simulink model "fuzzy_system"  (R2017a)
settings: Solver=VariableStepAuto  StartTime=0.0  StopTime=10  RelTol=1e-3
undefined symbols (not defined in the file or in its folder): tanks_level_system
libraries: simulink x1
settings Model: Creator=fredericovaz  LastModifiedBy=fredericovaz
settings SFSimCC: SimUseLocalCustomCode=on
settings RTWCC: RTWUseLocalCustomCode=on

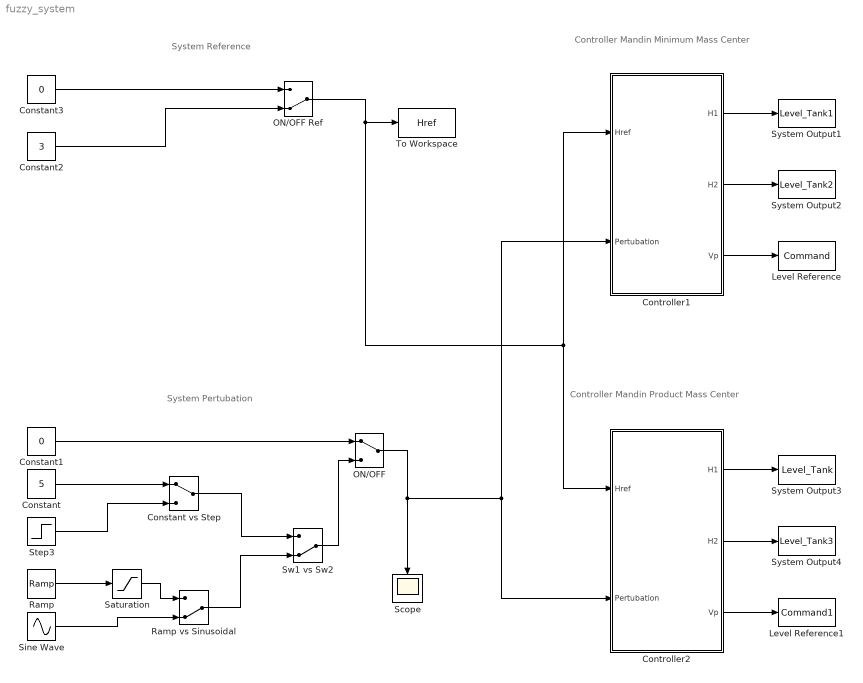
== system fuzzy_system ==
  note: Controller Mandin Minimum Mass Center
  note: Controller Mandin Product Mass Center
  note: System Pertubation
  note: System Reference
  Constant : Constant  Value=5
  Constant vs Step : ManualSwitch
  Constant1 : Constant  Value=0
  Constant2 : Constant  Value=3
  Constant3 : Constant  Value=0
  Controller1 : Subsystem
  Controller2 : Subsystem
  Level Reference : ToWorkspace  VariableName=Command  SaveFormat=Timeseries  SampleTime=-1
  Level Reference1 : ToWorkspace  VariableName=Command1  SaveFormat=Timeseries  SampleTime=-1
  ON/OFF : ManualSwitch
  ON/OFF Ref : ManualSwitch  CurrentSetting=0
  Ramp : simulink/Sources/Ramp  slope=2  start=60  X0=0
  Ramp vs Sinusoidal : ManualSwitch  CurrentSetting=0
  Saturation : Saturate  UpperLimit=5  LowerLimit=0
  Scope : Scope
  Sine Wave : Sin  Amplitude=5  Frequency=20  SampleTime=0
  Step3 : Step  Time=60  After=5  SampleTime=0
  Sw1 vs Sw2 : ManualSwitch  CurrentSetting=0
  System Output1 : ToWorkspace  VariableName=Level_Tank1  SaveFormat=Timeseries  SampleTime=-1
  System Output2 : ToWorkspace  VariableName=Level_Tank2  SaveFormat=Timeseries  SampleTime=-1
  System Output3 : ToWorkspace  VariableName=Level_Tank  SaveFormat=Timeseries  SampleTime=-1
  System Output4 : ToWorkspace  VariableName=Level_Tank3  SaveFormat=Timeseries  SampleTime=-1
  To Workspace : ToWorkspace  VariableName=Href  SaveFormat=Timeseries  SampleTime=-1
  wires:
  ON/OFF Ref/1 -> Controller2/1(Href), Controller1/1(Href), To Workspace/1
  Controller1/2(H2) -> System Output2/1
  Controller1/3(Vp) -> Level Reference/1
  Controller1/1(H1) -> System Output1/1
  Controller2/3(Vp) -> Level Reference1/1
  Controller2/1(H1) -> System Output3/1
  Controller2/2(H2) -> System Output4/1
  ON/OFF/1 -> Scope/1, Controller1/2(Pertubation), Controller2/2(Pertubation)
  Saturation/1 -> Ramp vs Sinusoidal/1
  Constant/1 -> Constant vs Step/1
  Ramp vs Sinusoidal/1 -> Sw1 vs Sw2/2
  Constant vs Step/1 -> Sw1 vs Sw2/1
  Sine Wave/1 -> Ramp vs Sinusoidal/2
  Step3/1 -> Constant vs Step/2
  Ramp/1 -> Saturation/1
  Constant1/1 -> ON/OFF/1
  Sw1 vs Sw2/1 -> ON/OFF/2
  Constant3/1 -> ON/OFF Ref/1
  Constant2/1 -> ON/OFF Ref/2

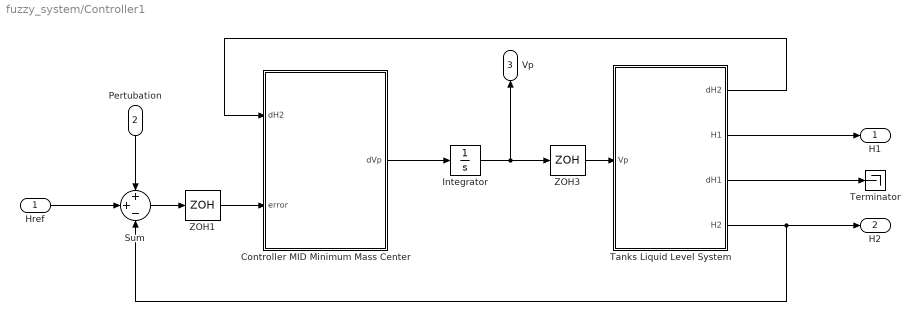
== system fuzzy_system/Controller1 ==
  Href : Inport
  Pertubation : Inport  Port=2
  Controller MID Minimum Mass Center : MATLAB Function  TreatAsAtomicUnit=on
  Integrator : Integrator
  Sum : Sum  Inputs=++-
  Tanks Liquid Level System : Subsystem
  Terminator : Terminator
  ZOH1 : ZeroOrderHold  SampleTime=1e-3
  ZOH3 : ZeroOrderHold  SampleTime=1e-3
  H1 : Outport
  H2 : Outport  Port=2
  Vp : Outport  Port=3
  wires:
  Tanks Liquid Level System/4(H2) -> H2/1, Sum/3
  Tanks Liquid Level System/1(dH2) -> Controller MID Minimum Mass Center/1(dH2)
  Tanks Liquid Level System/2(H1) -> H1/1
  ZOH3/1 -> Tanks Liquid Level System/1(Vp)
  Integrator/1 -> Vp/1, ZOH3/1
  Controller MID Minimum Mass Center/1(dVp) -> Integrator/1
  Tanks Liquid Level System/3("dH1 ") -> Terminator/1
  Sum/1 -> ZOH1/1
  Pertubation/1 -> Sum/1
  Href/1 -> Sum/2
  ZOH1/1 -> Controller MID Minimum Mass Center/2(error)

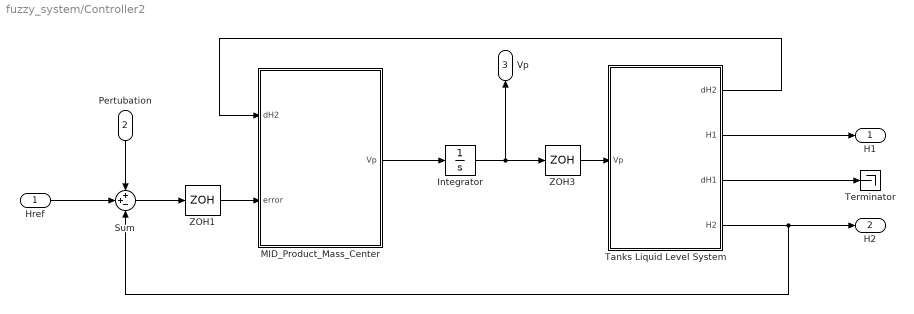
== system fuzzy_system/Controller2 ==
  Href : Inport
  Pertubation : Inport  Port=2
  Integrator : Integrator
  MID_Product_Mass_Center : MATLAB Function  TreatAsAtomicUnit=on
  Sum : Sum  Inputs=++-
  Tanks Liquid Level System : Subsystem
  Terminator : Terminator
  ZOH1 : ZeroOrderHold  SampleTime=1e-3
  ZOH3 : ZeroOrderHold  SampleTime=1e-3
  H1 : Outport
  H2 : Outport  Port=2
  Vp : Outport  Port=3
  wires:
  Tanks Liquid Level System/4(H2) -> H2/1, Sum/3
  Tanks Liquid Level System/1(dH2) -> MID_Product_Mass_Center/1(dH2)
  Tanks Liquid Level System/2(H1) -> H1/1
  ZOH3/1 -> Tanks Liquid Level System/1(Vp)
  ZOH1/1 -> MID_Product_Mass_Center/2(error)
  Sum/1 -> ZOH1/1
  Integrator/1 -> Vp/1, ZOH3/1
  MID_Product_Mass_Center/1(Vp) -> Integrator/1
  Tanks Liquid Level System/3("dH1 ") -> Terminator/1
  Href/1 -> Sum/2
  Pertubation/1 -> Sum/1

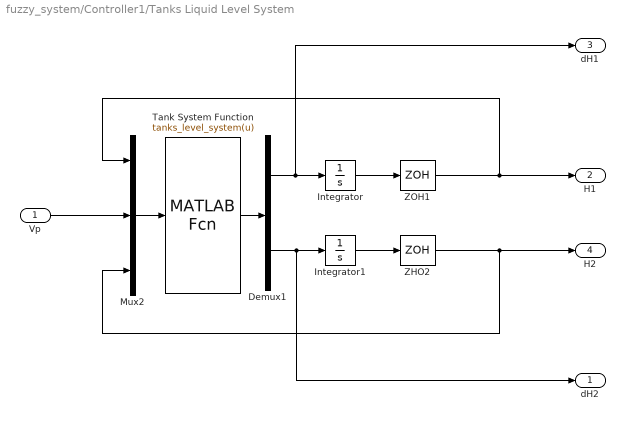
== system fuzzy_system/Controller1/Tanks Liquid Level System ==
  Vp : Inport
  Demux1 : Demux  Outputs=2
  Integrator : Integrator
  Integrator1 : Integrator
  Mux2 : Mux  Inputs=3
  Tank System Function : MATLABFcn  MATLABFcn=tanks_level_system(u)  OutputDimensions=2
  ZHO2 : ZeroOrderHold  SampleTime=1e-3
  ZOH1 : ZeroOrderHold  SampleTime=1e-3
  dH2 : Outport
  H1 : Outport  Port=2
  "dH1 " : Outport  Port=3
  H2 : Outport  Port=4
  wires:
  Demux1/2 -> Integrator1/1, dH2/1
  Integrator1/1 -> ZHO2/1
  Vp/1 -> Mux2/2
  ZHO2/1 -> H2/1, Mux2/3
  Integrator/1 -> ZOH1/1
  Tank System Function/1 -> Demux1/1
  ZOH1/1 -> H1/1, Mux2/1
  Demux1/1 -> Integrator/1, "dH1 "/1
  Mux2/1 -> Tank System Function/1

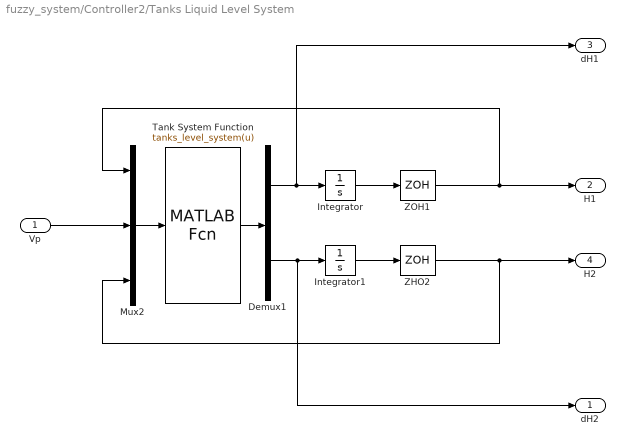
== system fuzzy_system/Controller2/Tanks Liquid Level System ==
  Vp : Inport
  Demux1 : Demux  Outputs=2
  Integrator : Integrator
  Integrator1 : Integrator
  Mux2 : Mux  Inputs=3
  Tank System Function : MATLABFcn  MATLABFcn=tanks_level_system(u)  OutputDimensions=2
  ZHO2 : ZeroOrderHold  SampleTime=1e-3
  ZOH1 : ZeroOrderHold  SampleTime=1e-3
  dH2 : Outport
  H1 : Outport  Port=2
  "dH1 " : Outport  Port=3
  H2 : Outport  Port=4
  wires:
  Demux1/2 -> Integrator1/1, dH2/1
  Integrator1/1 -> ZHO2/1
  Vp/1 -> Mux2/2
  ZHO2/1 -> H2/1, Mux2/3
  Integrator/1 -> ZOH1/1
  Tank System Function/1 -> Demux1/1
  ZOH1/1 -> H1/1, Mux2/1
  Demux1/1 -> Integrator/1, "dH1 "/1
  Mux2/1 -> Tank System Function/1

== matlab function fuzzy_system/Controller2/MID_Product_Mass_Center ==
  data: dH2 input; error input; Vp output

%%

function Vp  = fcn(dH2, error)


Vp = error;


end

== matlab function fuzzy_system/Controller1/Controller MID Minimum Mass Center ==
  data: dH2 input; dVp output; error input

function dVp  = fcn(dH2, error)
%% Controller Minimum Mass Center Function
%   - Triangular Diffuser
%   - Motor de Inferência de Mínimo
%   - Desdifusor por Centro de Massa

%--------------------------------------------------------------------------
% Diffusers and Trust Values
%--------------------------------------------------------------------------
% Calculo dos valores de pertença em cada conjundo difuso


% Error between Reference (Href) and Tank2 Level (H2) 
error_MH = error_MuchHigher(error);                     % Much Higher
error_M = error_Higher(error);                          % Higher 
error_C = error_Close(error);                           % Close
error_L = error_Lower(error);                           % Lower
error_ML = error_MuchLower(error);                      % Much Lower


% Tank2 Level Variation: dH2 
dH2_DF = dH2_DownFast(dH2);                             % Down Fast
dH2_D = dH2_Down(dH2);                                  % Down
dH2_S = dH2_Slow(dH2);                                  % Slow
dH2_U = dH2_Up(dH2);                                    % Up
dH2_UF = dH2_UpFast(dH2);                               % Up Fast


%--------------------------------------------------------------------------
% IF THEN Rules
%--------------------------------------------------------------------------
rule01 = min( error_MH, dH2_DF ); 
rule02 = min( error_MH, dH2_D );
rule03 = min( error_MH, dH2_S );
rule04 = min( error_MH, dH2_U );
rule05 = min( error_MH, dH2_UF );

rule06 = min( error_H, dH2_DF );
rule07 = min( error_H, dH2_D );
rule08 = min( error_H, dH2_S );
rule09 = min( error_H, dH2_U );
rule10 = min( error_H, dH2_UF );

rule11 = min( error_C, dH2_DF );
rule12 = min( error_C, dH2_D );
rule13 = min( error_C, dH2_S );
rule14 = min( error_C, dH2_U );
rule15 = min( error_C, dH2_UF );

rule16 = min( error_L, dH2_DF );
rule17 = min( error_L, dH2_D );
rule18 = min( error_L, dH2_S );
rule19 = min( error_L, dH2_U );
rule20 = min( error_L, dH2_UF );

rule21 = min( error_ML, dH2_DF );
rule22 = min( error_ML, dH2_D );
rule23 = min( error_ML, dH2_S );
rule24 = min( error_ML, dH2_U );
rule25 = min( error_ML, dH2_UF );

%--------------------------------------------------------------------------
% MID Mamdani min
%--------------------------------------------------------------------------
% Motor de Inferência Difusa de Mínimo onde
% A t-norma escolhida é o min
% A s-norma escolha é o max

dVp_DecM = max([rule11 rule12 rule13 rule14 rule17]);  % Large Decrements
dVp_Dec = max([rule10 rule15]);                        % Decrements 
dVp_M = max([rule06 rule09 rule16]);                   % Keeps
dVp_Inc = max([rule05 rule08]);                        % Increase
dVp_IncM = max([rule01 rule02 rule03 rule04 rule07]);  % Large Increase



%--------------------------------------------------------------------------
% Difuzzifier: Desdifusor Centro Gravidade
%--------------------------------------------------------------------------
% Onde in é a saída do MID e o x usado é o intervalo do universo de discurso de dV
% discretizado. Ou seja, x = -k:0.01:k, em que k é definido no ficheiro do
% controlador que junta as peças que constituem o mesmo. Neste caso, k = 4.

% dv = Desdifusor_Centro_Gravidade(cds, x);

k = 4;
x = -k:0.01:k;

dVp = sum(x.*in)/sum(in);


Vp = error;

end



%--------------------------------------------------------------------------
% Init
%--------------------------------------------------------------------------

% dH2_ = zeros(5);
% error_ = zeros(5);


% % Error between -100 and 100
% error = ((Href - H2)/100)*100;
% 
% % Normalized dH2
% dH2_norm = dH2/abs(error);


%--------------------------------------------------------------------------
% Diffusers
%--------------------------------------------------------------------------

% Tank2 Level Variation: dH2 

% [ dif_MU,dif_U,dif_A,dif_D,dif_MD ] = fuzzy1();
% 
% % More UP
% % UP
% % Slow
% % Down
% % More Down
% 
% % Voltage Motor Variation: dVp
% [ DM, dif_D, M, I, IM] = fuzzy2();


%--------------------------------------------------------------------------
% Trust Values
%--------------------------------------------------------------------------
